simulink model "MSAPOnduleurCommande"  (R2022b)
settings: Solver=ode1  StartTime=0.0  StopTime=10  FixedStep=1e-5  RelTol=1e-5  AbsTol=1e-5
values from neighbouring files (symbols this model uses):
  A = [0 -Lq  ; Ld 0 ]    [PARAMATRESMSAP.m]
  F = 0.0014    [PARAMATRESMSAP.m]
  J = 0.02    [PARAMATRESMSAP.m]
  Kid = 5109.49    [PARAMATRESMSAP.m]
  Kim = 5.0175    [PARAMATRESMSAP.m]
  Kiq = 5054.15    [PARAMATRESMSAP.m]
  Kpd = 27.4    [PARAMATRESMSAP.m]
  Kpm = 0.3986    [PARAMATRESMSAP.m]
  Kpq = 55.4    [PARAMATRESMSAP.m]
  L = [Ld 0 ; 0 Lq ]    [PARAMATRESMSAP.m]
  Ld = 2.8e-3    (= 0.0028)    [PARAMATRESMSAP.m]
  Lq = 1.4e-3    (= 0.0014)    [PARAMATRESMSAP.m]
  P = 4    [PARAMATRESMSAP.m]
  pf = 0.2    [PARAMATRESMSAP.m]
  phif = [0 ; pf]    [PARAMATRESMSAP.m]
  R = [Rs 0; 0 Rs ]    [PARAMATRESMSAP.m]
  Td = 1/fd    (= 0.0002)    [PARAMATRESMSAP.m]
  VDC = 600    [PARAMATRESMSAP.m]
  VP = VDC/2    (= 300)    [PARAMATRESMSAP.m]
libraries: simulink x1
settings Model: Creator=ZinouAb  LastModifiedBy=ZinouAb

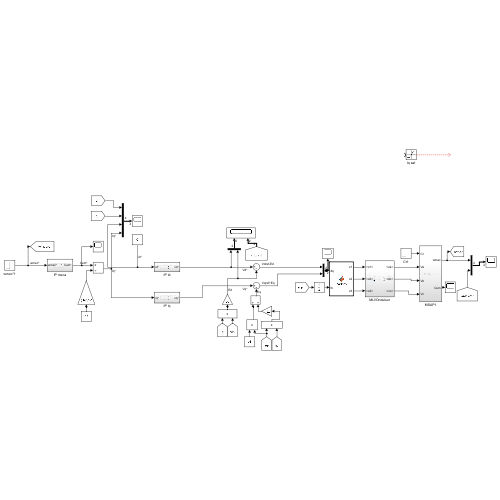
[thumbnail: Simulink's stored preview of the top-level diagram]
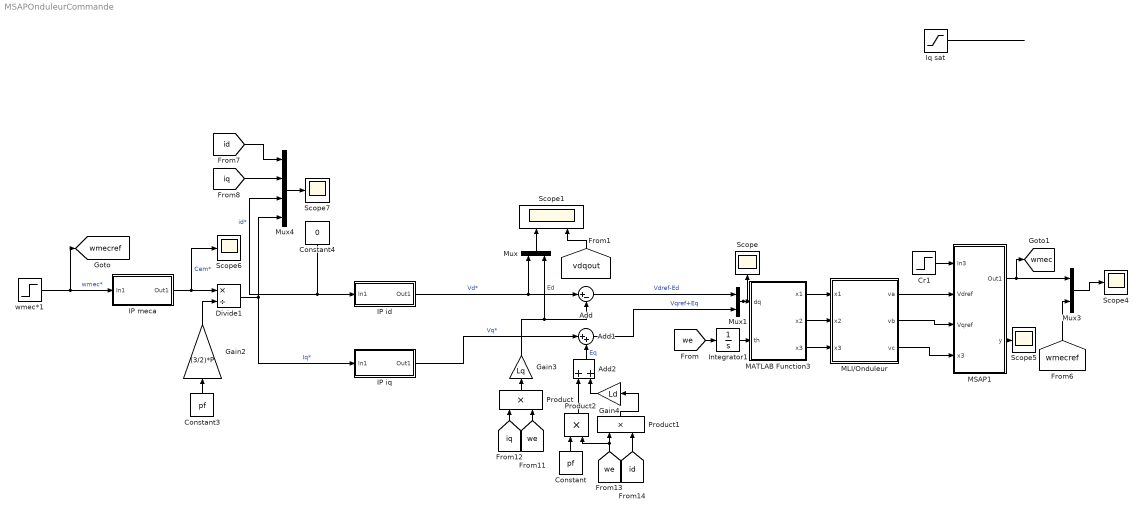
== system MSAPOnduleurCommande ==
  Add : Sum  Inputs=|+-
  Add1 : Sum  Inputs=|++
  Add2 : Sum
  Constant : Constant  Value=pf
  Constant3 : Constant  Value=pf
  Constant4 : Constant  Value=0
  Cr1 : Step  Time=6  Before=0.5  After=3  SampleTime=0
  Divide1 : Product  Inputs=*/
  Gain2 : Gain  Gain=(3/2)*P
  Gain3 : Gain  Gain=Lq
  Gain4 : Gain  Gain=Ld
  IP id : Subsystem
  IP iq : Subsystem
  IP meca : Subsystem
  Integrator1 : Integrator
  Iq sat : Saturate  UpperLimit=20  LowerLimit=-20
  MATLAB Function3 : MATLAB Function  TreatAsAtomicUnit=on
  MLI/Onduleur : Subsystem
  MSAP1 : Subsystem
  Mux : Mux  Inputs=2
  Mux1 : Mux  Inputs=2
  Mux3 : Mux  Inputs=2
  Mux4 : Mux
  Product : Product
  Product1 : Product
  Product2 : Product
  Scope{,4..7} (5 alike) : Scope
  Scope1 : Scope  NumInputPorts=2
  wmec*1 : Step  Time=4  After=314  SampleTime=0
  tag scope: wmec=global, wmecref=global
  wires:
  [we] -> Product/2
  MSAP1/1(Out1) -> [wmec], Mux3/1
  MSAP1/2(y) -> Scope5/1
  Gain4/1 -> Add2/2
  Constant/1 -> Product2/1
  [we] -> Product2/2, Product1/1
  Product2/1 -> Add2/1
  Product/1 -> Gain3/1
  IP iq/1(Out1) -> Add1/1  "Vq*"
  Add2/1 -> Add1/2  "Eq"
  Gain3/1 -> Mux/2, Add/2  "Ed"
  Product1/1 -> Gain4/1
  [id] -> Product1/2
  [iq] -> Product/1
  Mux4/1 -> Scope7/1
  Constant3/1 -> Gain2/1
  Mux3/1 -> Scope4/1
  IP id/1(Out1) -> Mux/1, Add/1  "Vd*"
  Constant4/1 -> IP id/1(In1), Mux4/3  "id*"
  [wmecref] -> Mux3/2
  [id] -> Mux4/1
  Divide1/1 -> IP iq/1(In1), Mux4/4  "Iq*"
  wmec*1/1 -> IP meca/1(In1), [wmecref]  "wmec*"
  IP meca/1(Out1) -> Divide1/1, Scope6/1  "Cem*"
  [iq] -> Mux4/2
  Gain2/1 -> Divide1/2
  Cr1/1 -> MSAP1/1(In3)
  Add1/1 -> Mux1/2  "Vqref+Eq"
  Integrator1/1 -> MATLAB Function3/2(th)
  Add/1 -> Mux1/1  "Vdref-Ed"
  [we] -> Integrator1/1
  Mux1/1 -> MATLAB Function3/1(dq), Scope/1
  MLI/Onduleur/2(vb) -> MSAP1/3(Vqref)
  MLI/Onduleur/1(va) -> MSAP1/2(Vdref)
  MLI/Onduleur/3(vc) -> MSAP1/4(x3)
  MATLAB Function3/1(x1) -> MLI/Onduleur/1(x1)
  MATLAB Function3/2(x2) -> MLI/Onduleur/2(x2)
  MATLAB Function3/3(x3) -> MLI/Onduleur/3(x3)
  Iq sat/1 -> ?
  Mux/1 -> Scope1/1
  [vdqout] -> Scope1/2

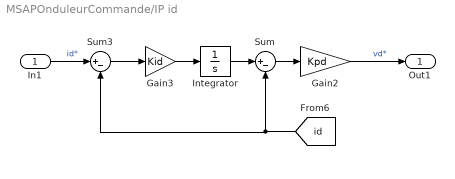
== system MSAPOnduleurCommande/IP id ==
  In1 : Inport
  Gain2 : Gain  Gain=Kpd
  Gain3 : Gain  Gain=Kid
  Integrator : Integrator
  Sum : Sum  Inputs=|+-
  Sum3 : Sum  Inputs=|+-
  Out1 : Outport
  wires:
  Integrator/1 -> Sum/1
  [id] -> Sum3/2, Sum/2
  Sum/1 -> Gain2/1
  Gain2/1 -> Out1/1  "vd*"
  Gain3/1 -> Integrator/1
  Sum3/1 -> Gain3/1
  In1/1 -> Sum3/1  "id*"

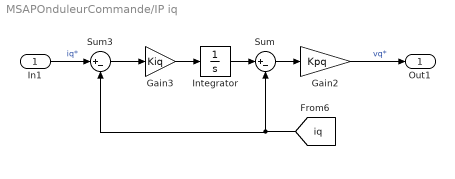
== system MSAPOnduleurCommande/IP iq ==
  In1 : Inport
  Gain2 : Gain  Gain=Kpq
  Gain3 : Gain  Gain=Kiq
  Integrator : Integrator
  Sum : Sum  Inputs=|+-
  Sum3 : Sum  Inputs=|+-
  Out1 : Outport
  wires:
  Integrator/1 -> Sum/1
  [iq] -> Sum3/2, Sum/2
  Sum/1 -> Gain2/1
  Gain2/1 -> Out1/1  "vq*"
  Gain3/1 -> Integrator/1
  Sum3/1 -> Gain3/1
  In1/1 -> Sum3/1  "iq*"

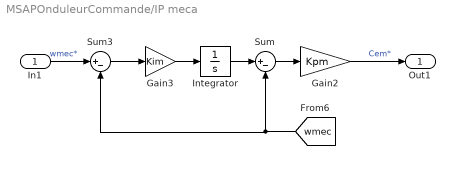
== system MSAPOnduleurCommande/IP meca ==
  In1 : Inport
  Gain2 : Gain  Gain=Kpm
  Gain3 : Gain  Gain=Kim
  Integrator : Integrator
  Sum : Sum  Inputs=|+-
  Sum3 : Sum  Inputs=|+-
  Out1 : Outport
  wires:
  Integrator/1 -> Sum/1
  [wmec] -> Sum3/2, Sum/2
  Sum/1 -> Gain2/1
  Gain2/1 -> Out1/1  "Cem*"
  Gain3/1 -> Integrator/1
  Sum3/1 -> Gain3/1
  In1/1 -> Sum3/1  "wmec*"

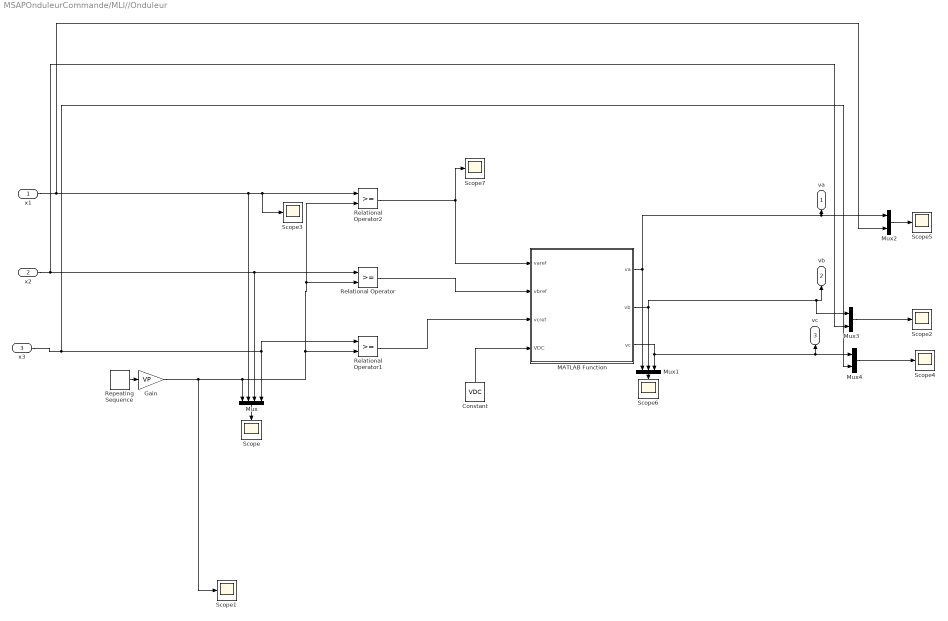
== system MSAPOnduleurCommande/MLI//Onduleur ==
  x1 : Inport
  x2 : Inport  Port=2
  x3 : Inport  Port=3
  Constant : Constant  Value=VDC
  Gain : Gain  Gain=VP
  MATLAB Function : MATLAB Function  TreatAsAtomicUnit=on
  Mux : Mux
  Mux1 : Mux  Inputs=3
  Mux2 : Mux  Inputs=2
  Mux3 : Mux  Inputs=2
  Mux4 : Mux  Inputs=2
  Relational Operator : RelationalOperator  OutDataTypeStr=boolean  RndMeth=Simplest  InputSameDT=off
  Relational Operator1 : RelationalOperator  OutDataTypeStr=boolean  RndMeth=Simplest  InputSameDT=off
  Relational Operator2 : RelationalOperator  OutDataTypeStr=boolean  RndMeth=Simplest  InputSameDT=off
  Repeating Sequence : simulink/Sources/Repeating Sequence  rep_seq_t=[0 0.5 1].*Td  rep_seq_y=[-1 1 -1]
  Scope{,1..7} (8 alike) : Scope
  va : Outport
  vb : Outport  Port=2
  vc : Outport  Port=3
  wires:
  Mux/1 -> Scope/1
  Gain/1 -> Scope1/1, Mux/1, Relational Operator1/2, Relational Operator/2, Relational Operator2/2
  Relational Operator/1 -> MATLAB Function/2(vbref)
  Relational Operator1/1 -> MATLAB Function/3(vcref)
  Relational Operator2/1 -> Scope7/1, MATLAB Function/1(varef)
  MATLAB Function/1(va) -> va/1, Mux2/1, Mux1/1
  Constant/1 -> MATLAB Function/4(VDC)
  Mux1/1 -> Scope6/1
  Mux2/1 -> Scope5/1
  MATLAB Function/2(vb) -> vb/1, Mux3/1, Mux1/2
  Mux3/1 -> Scope2/1
  MATLAB Function/3(vc) -> Mux1/3, vc/1, Mux4/1
  Mux4/1 -> Scope4/1
  x1/1 -> Mux2/2, Mux/2, Relational Operator2/1, Scope3/1
  x2/1 -> Mux3/2, Relational Operator/1, Mux/3
  x3/1 -> Mux4/2, Relational Operator1/1, Mux/4
  Repeating Sequence/1 -> Gain/1

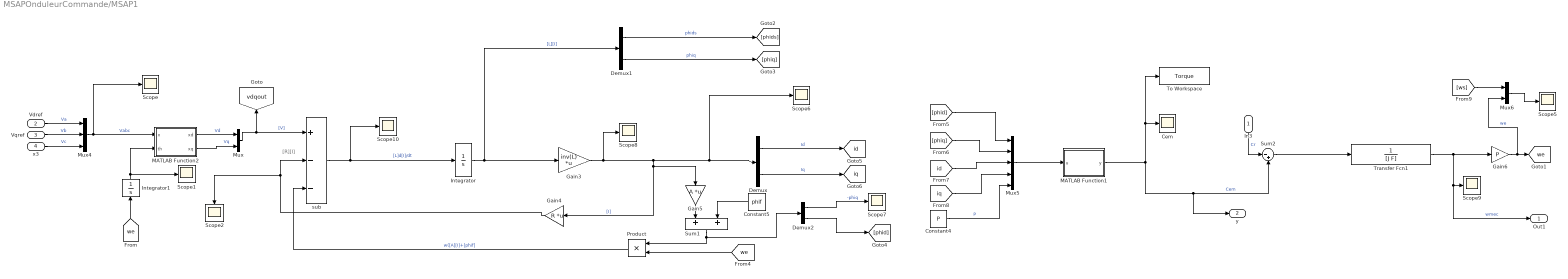
== system MSAPOnduleurCommande/MSAP1 ==
  note: [R][I]
  In3 : Inport
  Vdref : Inport  Port=2
  Vqref : Inport  Port=3
  x3 : Inport  Port=4
  Cem : Scope
  Constant4 : Constant  Value=P
  Constant5 : Constant  Value=phif
  Demux : Demux  Outputs=2
  Demux1 : Demux  Outputs=2
  Demux2 : Demux  Outputs=2
  Gain3 : Gain  Gain=inv(L)  Multiplication=Matrix(K*u)
  Gain4 : Gain  Gain=R  Multiplication=Matrix(K*u)
  Gain5 : Gain  Gain=A  Multiplication=Matrix(K*u)
  Gain6 : Gain  Gain=P
  Integrator : Integrator
  Integrator1 : Integrator
  MATLAB Function1 : MATLAB Function  TreatAsAtomicUnit=on
  MATLAB Function2 : MATLAB Function  TreatAsAtomicUnit=on
  Mux : Mux  Inputs=2
  Mux4 : Mux  Inputs=3
  Mux5 : Mux  Inputs=5
  Mux6 : Mux  Inputs=2
  Product : Product
  Scope{,1..2,5..10} (9 alike) : Scope
  Sum1 : Sum
  Sum2 : Sum  Inputs=|-+
  To Workspace : ToWorkspace  VariableName=Torque  SaveFormat=Timeseries  SampleTime=-1
  Transfer Fcn1 : TransferFcn  Denominator=[J F]
  sub : Sum  Inputs=+--
  Out1 : Outport
  y : Outport  Port=2
  tag scope: id=global, iq=global, vdqout=global, we=global
  wires:
  sub/1 -> Scope10/1, Integrator/1  "[L]d[I]/dt"
  MATLAB Function1/1(y) -> To Workspace/1, Cem/1, y/1, Sum2/2  "Cem"
  Product/1 -> sub/3  "w([A][I]+[phif]"
  Sum2/1 -> Transfer Fcn1/1
  Transfer Fcn1/1 -> Out1/1, Scope9/1, Gain6/1  "wmec"
  Vdref/1 -> Mux4/1  "Va"
  Gain4/1 -> Scope2/1, sub/2
  Gain6/1 -> Mux6/2, [we]  "we"
  Demux/2 -> [iq]  "Iq"
  Sum1/1 -> Product/1, Demux2/1
  Demux1/2 -> [phiq]  "phiq"
  Integrator/1 -> Gain3/1, Demux1/1  "[L][I]"
  Mux6/1 -> Scope5/1
  Constant4/1 -> Mux5/5  "P"
  Demux/1 -> [id]  "Id"
  [we] -> Product/2
  Gain5/1 -> Sum1/1
  Gain3/1 -> Gain4/1, Gain5/1, Scope6/1, Demux/1, Scope8/1  "[I]"
  Vqref/1 -> Mux4/2  "Vb"
  Mux5/1 -> MATLAB Function1/1(u)
  In3/1 -> Sum2/1  "Cr"
  Constant5/1 -> Sum1/2
  [id] -> Mux5/3
  [iq] -> Mux5/4
  Demux2/2 -> [phid]
  Demux2/1 -> Scope7/1  "-phiq"
  Mux/1 -> [vdqout], sub/1  "[V]"
  Demux1/1 -> [phids]  "phids"
  [phid] -> Mux5/1
  [phiq] -> Mux5/2
  [ws] -> Mux6/1
  x3/1 -> Mux4/3  "Vc"
  Mux4/1 -> Scope/1, MATLAB Function2/1(x)  "Vabc"
  MATLAB Function2/1(xd) -> Mux/1  "Vd"
  MATLAB Function2/2(xq) -> Mux/2  "Vq"
  [we] -> Integrator1/1
  Integrator1/1 -> Scope1/1, MATLAB Function2/2(th)

== matlab function MSAPOnduleurCommande/MATLAB Function3 ==
  data: dq input; x1 output; x2 output; x3 output; th input
function [x1,x2,x3]= Parkinv(dq,th)
parkinv = [ cos(th),           -sin(th); 
          cos(th-2*pi/3), -sin(th-2*pi/3); 
          cos(th+2*pi/3), -sin(th+2*pi/3)];
temp = parkinv * [dq];
x1=temp(1);
x2=temp(2);
x3=temp(3);

== matlab function MSAPOnduleurCommande/MLI//Onduleur/MATLAB Function ==
  data: varef input; vbref input; vcref input; VDC input; va output; vb output; vc output
function [va,vb,vc]= OnduleurOut(varef,vbref,vcref,VDC)
varef=double(varef);
vbref=double(vbref);
vcref=double(vcref);
va=(2*varef-vbref-vcref)*(VDC/3);
vb=(2*vbref-varef-vcref)*(VDC/3);
vc=(2*vcref-vbref-varef)*(VDC/3);

== matlab function MSAPOnduleurCommande/MSAP1/MATLAB Function1 ==
  data: u input; y output
function y = CEM(u)

y =(3/2)*u(5)*(u(1)*u(4)-u(2)*u(3));

== matlab function MSAPOnduleurCommande/MSAP1/MATLAB Function2 ==
  data: x input; xd output; xq output; th input
function [xd,xq] = Park(x,th)
% vd=(2/3)*(u1*cos(th)+u2*cos(th-2*pi/3)+u3*cos(th+2*pi/3));
% vq=(2/3)*(-u1*sin(th)-u2*sin(th-2*pi/3)-u3*sin(th+2*pi/3));
P=(2/3)*[ cos(th) cos(th-2*pi/3) cos(th+2*pi/3);
         -sin(th) -sin(th-2*pi/3) -sin(th+2*pi/3)  ];
prod=P*x;
xd=prod(1);
xq=prod(2);
